simulink model "csdesigner_Preg_14v"  (R2014a)
settings: Solver=ode45  SolverMode=SingleTasking  StartTime=0.0  StopTime=10  RelTol=1e-3
values from neighbouring files (symbols this model uses):
  delay = 0.001    [init_regul.m]
  delta = 4e-6    (= 4e-06)    [main.m]
  Ecz = 0    [init_regul.m]
  F2 = a*mass*g/(a+b)    (= 15.4982642891)    [main.m]
  g = 9.81    [main.m]
  h0 = 75e-6    (= 7.5e-05)    [main.m]
  KAD = 0    [init_regul.m]
  Kpb = 5.5    [init_regul.m]
  Kps = (Vmax-Vmin)/(Hmax-Hmin)    (= 1666.66666667)    [main.m]
  Ksv = 30    [main.m]
  Kx = 1    [init_regul.m]
  Ky = 1    [init_regul.m]
  mm = F2/g    (= 1.57984345455)    [main.m]
  nu = 1/h0    (= 13333.3333333)    [main.m]
  omega = n_rpm*2*pi/60    (= 293.215314335)    [main.m]
  tau = 0.12    [main.m]
  Ts = 1/fs    (= 0.001)    [main.m]
  Ux0 = 3    [init_regul.m]
  Uy0 = 3    [init_regul.m]
  Wx = 5    [init_regul.m]
  Wy = 5    [init_regul.m]
  xeq = x(end,1)    [main.m]
  yeq = x(end,3)    [main.m]
undefined symbols (not defined in the file or in its folder): DiscIntNeverNeededParam
libraries: neural x162, dspmathops x4, simulink x3
(part 1 of 4)
settings Model: CovMetricSettings=dwe  CovHtmlReporting=off  covSaveCumulativeToWorkspaceVar=off  CovSaveSingleToWorkspaceVar=off  CovExternalEMLEnable=on  CovSFcnEnable=on  Creator=Alexander  LastModifiedBy=Юрий
settings DataIOCC: LimitDataPoints=off  SaveFormat=StructureWithTime  ReturnWorkspaceOutputs=on
settings DebuggingCC: MergeDetectMultiDrivingBlocksExec=error  SolverPrmCheckMsg=none  FrameProcessingCompatibilityMsg=error  SFUnexpectedBacktrackingDiag=error  SFNoUnconditionalDefaultTransitionDiag=error
settings HardwareCC: ProdBitPerPointer=64  ProdLargestAtomicFloat=Float  ProdIntDivRoundTo=Zero  ProdEndianess=LittleEndian  ProdHWDeviceType=Specified
settings ModelReferenceCC: PropagateSignalLabelsOutOfModel=on
settings SFSimCC: SimUseLocalCustomCode=on
settings RTWCC: RTWUseLocalCustomCode=on
settings GRTTargetCC: TargetLangStandard=C99 (ISO)

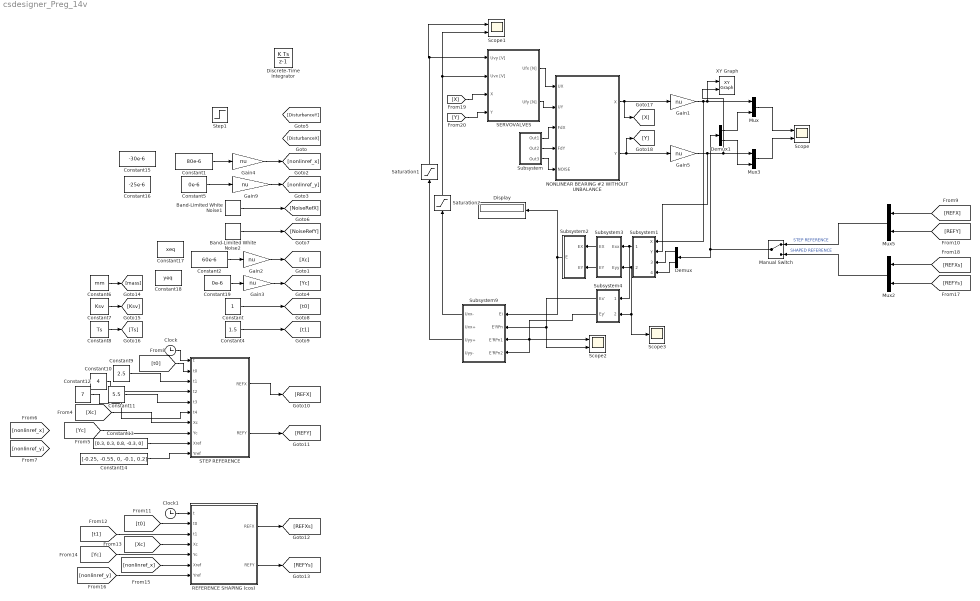
== system csdesigner_Preg_14v ==
  Band-Limited White Noise1 : simulink/Sources/Band-Limited White Noise  Cov=n_pow  Ts=Ts  seed=[23341]
  Band-Limited White Noise2 : simulink/Sources/Band-Limited White Noise  Cov=n_pow  Ts=1.1*Ts  seed=[23341]
  Clock : Clock
  Clock1 : Clock
  Constant : Constant
  Constant1 : Constant  Value=80e-6
  Constant10 : Constant  Value=4
  Constant11 : Constant  Value=5.5
  Constant12 : Constant  Value=7
  Constant13 : Constant  Value=[0.3, 0.3, 0.8, -0.3, 0]
  Constant14 : Constant  Value=[-0.25, -0.55, 0, -0.1, 0.2]
  Constant15 : Constant  Value=-30e-6
  Constant16 : Constant  Value=-25e-6
  Constant17 : Constant  Value=xeq
  Constant18 : Constant  Value=yeq
  Constant19 : Constant  Value=0e-6
  Constant2 : Constant  Value=60e-6
  Constant4 : Constant  Value=1.5
  Constant5 : Constant  Value=0e-6
  Constant6 : Constant  Value=mm
  Constant7 : Constant  Value=Ksv
  Constant8 : Constant  Value=Ts
  Constant9 : Constant  Value=2.5
  Demux : Demux  Outputs=2
  Demux1 : Demux  Outputs=2
  Discrete-Time Integrator : DiscreteIntegrator  InitialConditionSetting=State (most efficient)  SampleTime=-1  ICPrevOutput=DiscIntNeverNeededParam  ICPrevScaledInput=DiscIntNeverNeededParam
  Display : Display
  Gain{1..5,9} (6 alike) : Gain  Gain=nu
  Manual Switch : ManualSwitch
  Mux{,2..3,5} (4 alike) : Mux  Inputs=2
  NONLINEAR BEARING #2 WITHOUT UNBALANCE : Subsystem
  REFERENCE SHAPING (cos) : MATLAB Function  TreatAsAtomicUnit=on
      settings: PermitHierarchicalResolution=ParametersOnly
  SERVOVALVES : Subsystem
  STEP REFERENCE : MATLAB Function  TreatAsAtomicUnit=on
      settings: PermitHierarchicalResolution=ParametersOnly
  Saturation1 : Saturate  UpperLimit=10  LowerLimit=0
  Saturation2 : Saturate  UpperLimit=10  LowerLimit=0
  Scope : Scope  NumInputPorts=2
      settings: TimeRange=10  TickLabels=on  ShowLegends=on  MaxDataPoints=5000  SaveToWorkspace=off  SaveName=ScopeData  YMin=-0.50237~-0.65259  YMax=0.94471~0.29473  SampleTime=-1
  Scope1 : Scope  NumInputPorts=2
      settings: TimeRange=auto  MaxDataPoints=5000  SaveToWorkspace=off  YMin=-1.17846~-5  YMax=11.24205~5  SampleTime=-1
  Scope2 : Scope  NumInputPorts=2
      settings: TimeRange=auto  MaxDataPoints=5000  SaveToWorkspace=off  SaveName=ScopeData2  YMin=-1.34323~-5  YMax=0.95187~5  SampleTime=-1
  Scope3 : Scope
      settings: TimeRange=auto  MaxDataPoints=5000  SaveToWorkspace=off  SaveName=ScopeData2  YMin=-0.64553  YMax=0.24338  SampleTime=-1
  Step1 : Step  After=-10  SampleTime=0
  Subsystem : Subsystem
  Subsystem1 : Subsystem
  Subsystem2 : Subsystem
  Subsystem3 : Subsystem
  Subsystem4 : Subsystem
  Subsystem9 : Subsystem
  XY Graph : simulink/Sinks/XY Graph  xmin=-1  xmax=1  ymin=-1  ymax=1  st=-1
  wires:
  Constant7/1 -> [Ksv]
  [t0] -> STEP REFERENCE/2(t0)
  [nonlinref_y] -> REFERENCE SHAPING (cos)/7(Yref)
  [nonlinref_x] -> REFERENCE SHAPING (cos)/6(Xref)
  Constant8/1 -> [Ts]
  Constant6/1 -> [mass]
  Constant19/1 -> Gain3/1
  Mux5/1 -> Manual Switch/1  "STEP REFERENCE"
  [REFY] -> Mux5/2
  Clock1/1 -> REFERENCE SHAPING (cos)/1(t)
  Demux1/2 -> Mux3/2
  REFERENCE SHAPING (cos)/2(REFY) -> [REFYs]
  [REFX] -> Mux5/1
  Constant2/1 -> Gain2/1
  REFERENCE SHAPING (cos)/1(REFX) -> [REFXs]
  [Yc] -> REFERENCE SHAPING (cos)/5(Yc)
  Clock/1 -> STEP REFERENCE/1(t)
  [Xc] -> REFERENCE SHAPING (cos)/4(Xc)
  [t0] -> REFERENCE SHAPING (cos)/2(t0)
  Constant4/1 -> [t1]
  Gain3/1 -> [Yc]
  [REFXs] -> Mux2/1
  [t1] -> REFERENCE SHAPING (cos)/3(t1)
  [REFYs] -> Mux2/2
  [Xc] -> STEP REFERENCE/7(Xc)
  Mux2/1 -> Manual Switch/2  "SHAPED REFERENCE"
  Mux3/1 -> Scope/2
  Mux/1 -> Scope/1
  Manual Switch/1 -> Demux1/1, Demux/1
  STEP REFERENCE/2(REFY) -> [REFY]
  Gain4/1 -> [nonlinref_x]
  Gain2/1 -> [Xc]
  STEP REFERENCE/1(REFX) -> [REFX]
  Gain9/1 -> [nonlinref_y]
  [Yc] -> STEP REFERENCE/8(Yc)
  Constant5/1 -> Gain9/1
  Constant/1 -> [t0]
  NONLINEAR BEARING #2 WITHOUT UNBALANCE/1(X) -> [X], Gain1/1
  Band-Limited White Noise1/1 -> [NoiseRefX]
  Band-Limited White Noise2/1 -> [NoiseRefY]
  NONLINEAR BEARING #2 WITHOUT UNBALANCE/2(Y) -> [Y], Gain5/1
  Constant1/1 -> Gain4/1
  SERVOVALVES/1(Ufx [N]) -> NONLINEAR BEARING #2 WITHOUT UNBALANCE/1(UX)
  SERVOVALVES/2(Ufy [N]) -> NONLINEAR BEARING #2 WITHOUT UNBALANCE/2(UY)
  [X] -> SERVOVALVES/3(X)
  [Y] -> SERVOVALVES/4(Y)
  Gain1/1 -> Subsystem1/1(X), XY Graph/1, Mux/1
  Gain5/1 -> Subsystem1/2(Y), XY Graph/2, Mux3/1
  Subsystem/1(Out1) -> NONLINEAR BEARING #2 WITHOUT UNBALANCE/3(FdX)
  Subsystem/2(Out2) -> NONLINEAR BEARING #2 WITHOUT UNBALANCE/4(FdY)
  Subsystem/3(Out3) -> NONLINEAR BEARING #2 WITHOUT UNBALANCE/5(NOISE)
  Demux/1 -> Subsystem1/3(refX)
  Demux/2 -> Subsystem1/4(refY)
  Subsystem1/1(Exx) -> Subsystem4/1(Exx), Subsystem3/1(Exx)
  Subsystem3/1(EX) -> Subsystem2/1(EX)
  Subsystem1/2(Eyy) -> Scope3/1, Subsystem4/2(Eyy), Subsystem3/2(Eyy)
  Subsystem3/2(EY) -> Subsystem2/2(EY)
  Subsystem2/1(E) -> Subsystem9/1(Ei), Display/1
  Subsystem4/1(Ex') -> Subsystem9/2(E'RPn), Scope2/2
  Subsystem4/2(Ey') -> Subsystem9/4(E'RPn2), Scope2/1, Subsystem9/3(E'RPn1)
  Subsystem9/1(Uxx-) -> Saturation2/1
  Demux1/1 -> Mux/2
  Constant9/1 -> STEP REFERENCE/3(t1)
  Constant10/1 -> STEP REFERENCE/4(t2)
  Constant11/1 -> STEP REFERENCE/5(t3)
  Constant12/1 -> STEP REFERENCE/6(t4)
  Constant13/1 -> STEP REFERENCE/9(Xref)
  Constant14/1 -> STEP REFERENCE/10(Yref)
  Saturation1/1 -> Scope1/1, SERVOVALVES/1(Uvy [V])
  Saturation2/1 -> Scope1/2, SERVOVALVES/2(Uvx [V])
  Subsystem9/3(Uyy+) -> Saturation1/1

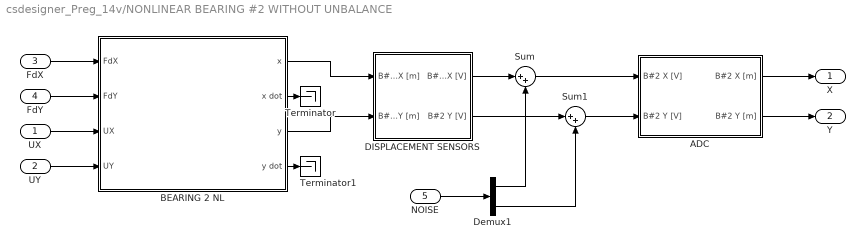
== system csdesigner_Preg_14v/NONLINEAR BEARING #2 WITHOUT UNBALANCE ==
  UX : Inport
  UY : Inport  Port=2
  FdX : Inport  Port=3
  FdY : Inport  Port=4
  NOISE : Inport  Port=5
  ADC : Subsystem
  BEARING 2 NL : Subsystem
  DISPLACEMENT SENSORS : Subsystem
  Demux1 : Demux  Outputs=2
  Sum : Sum  Inputs=|++
  Sum1 : Sum  Inputs=|++
  Terminator : Terminator
  Terminator1 : Terminator
  X : Outport
  Y : Outport  Port=2
  wires:
  BEARING 2 NL/3(y) -> DISPLACEMENT SENSORS/2(B#2 Y [m])
  BEARING 2 NL/1(x) -> DISPLACEMENT SENSORS/1(B#2 X [m])
  Demux1/2 -> Sum1/2
  NOISE/1 -> Demux1/1
  Demux1/1 -> Sum/2
  Sum1/1 -> ADC/2(B#2 Y [V])
  Sum/1 -> ADC/1(B#2 X [V])
  DISPLACEMENT SENSORS/1(B#2 X [V]) -> Sum/1
  DISPLACEMENT SENSORS/2(B#2 Y [V]) -> Sum1/1
  BEARING 2 NL/4(y dot) -> Terminator1/1
  BEARING 2 NL/2("x dot ") -> Terminator/1
  FdX/1 -> BEARING 2 NL/1(FdX)
  FdY/1 -> BEARING 2 NL/2(FdY)
  UY/1 -> BEARING 2 NL/4(UY)
  UX/1 -> BEARING 2 NL/3(UX)
  ADC/1(B#2 X [m]) -> X/1
  ADC/2(B#2 Y [m]) -> Y/1

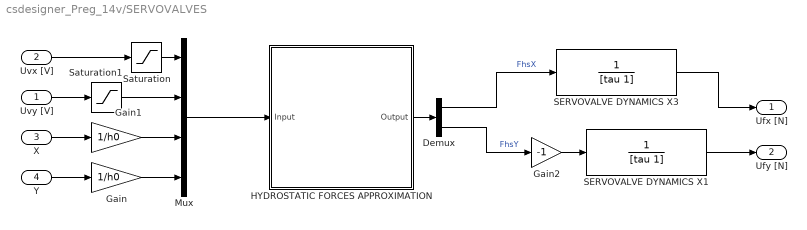
== system csdesigner_Preg_14v/SERVOVALVES ==
  Uvy [V] : Inport
  Uvx [V] : Inport  Port=2
  X : Inport  Port=3
  Y : Inport  Port=4
  Demux : Demux  Outputs=2
  Gain : Gain  Gain=1/h0
  Gain1 : Gain  Gain=1/h0
  Gain2 : Gain  Gain=-1
  HYDROSTATIC FORCES APPROXIMATION : Subsystem
      mask help: Function Fitting Neural Network
      mask Display: e = 0.06;c1 = [120 150 230]/255;c2 = ([120 150 230]+0)/383;c3 = ([120 150 230]+128)/383;patch([0 1 1 0],[0 0 1 1],c1);patch([0 1 1 1-e 1-e 0+e],[0 0 1 1-e 0+e 0+e],c2);patch([0 0 1 1-e 0+e 0+e],[0 1 1 1-e 1-e 0+e],c3);plot([0 1 1 0 0],[0 0 1 1 0]);fprintf('NNET');port_label('input',1,' Input');port_label('output',1,'Output ');
  Mux : Mux
  SERVOVALVE DYNAMICS X1 : TransferFcn  Numerator=1  Denominator=[tau 1]
  SERVOVALVE DYNAMICS X3 : TransferFcn  Numerator=1  Denominator=[tau 1]
  Saturation : Saturate  UpperLimit=10  LowerLimit=0
  Saturation1 : Saturate  UpperLimit=10  LowerLimit=0
  Ufx [N] : Outport
  Ufy [N] : Outport  Port=2
  wires:
  HYDROSTATIC FORCES APPROXIMATION/1(Output) -> Demux/1
  Demux/1 -> SERVOVALVE DYNAMICS X3/1  "FhsX"
  Demux/2 -> Gain2/1  "FhsY"
  Mux/1 -> HYDROSTATIC FORCES APPROXIMATION/1(Input)
  Y/1 -> Gain/1
  X/1 -> Gain1/1
  Uvy [V]/1 -> Saturation1/1
  Uvx [V]/1 -> Saturation/1
  Gain/1 -> Mux/4
  Gain1/1 -> Mux/3
  Saturation/1 -> Mux/1
  Saturation1/1 -> Mux/2
  Gain2/1 -> SERVOVALVE DYNAMICS X1/1
  SERVOVALVE DYNAMICS X3/1 -> Ufx [N]/1
  SERVOVALVE DYNAMICS X1/1 -> Ufy [N]/1

== system csdesigner_Preg_14v/Subsystem ==
  Mux1 : Mux  Inputs=2
  Out1 : Outport
  Out2 : Outport  Port=2
  Out3 : Outport  Port=3
  wires:
  [NoiseRefY] -> Mux1/2
  [NoiseRefX] -> Mux1/1
  [DisturbanceX] -> Out1/1
  [DisturbanceY] -> Out2/1
  Mux1/1 -> Out3/1

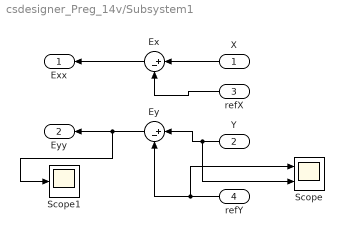
== system csdesigner_Preg_14v/Subsystem1 ==
  X : Inport
  Y : Inport  Port=2
  refX : Inport  Port=3
  refY : Inport  Port=4
  Ex : Sum  Inputs=|+-
  Ey : Sum  Inputs=|+-
  Scope : Scope  NumInputPorts=2
      settings: TimeRange=auto  MaxDataPoints=5000  SaveToWorkspace=off  SaveName=ScopeData3  YMin=-0.65259~-5  YMax=0.29473~5  SampleTime=-1
  Scope1 : Scope
      settings: TimeRange=auto  MaxDataPoints=5000  SaveToWorkspace=off  SaveName=ScopeData4  YMin=-0.64553  YMax=0.24338  SampleTime=-1
  Exx : Outport
  Eyy : Outport  Port=2
  wires:
  Ex/1 -> Exx/1
  Ey/1 -> Scope1/1, Eyy/1
  refX/1 -> Ex/2
  X/1 -> Ex/1
  Y/1 -> Scope/2, Ey/1
  refY/1 -> Scope/1, Ey/2

== system csdesigner_Preg_14v/Subsystem2 ==
  EX : Inport
  EY : Inport  Port=2
  Math Function : Math  Operator=square  SaturateOnIntegerOverflow=on
  Math Function1 : Math  Operator=square  SaturateOnIntegerOverflow=on
  Sqrt : Sqrt  SaturateOnIntegerOverflow=on
  Sum : Sum  Inputs=|++
  E : Outport
  wires:
  Sum/1 -> Sqrt/1
  Math Function1/1 -> Sum/2
  Math Function/1 -> Sum/1
  EY/1 -> Math Function1/1
  EX/1 -> Math Function/1
  Sqrt/1 -> E/1

== system csdesigner_Preg_14v/Subsystem3 ==
  Exx : Inport
  Eyy : Inport  Port=2
  Constant9 : Constant  Value=Ecz
  Sum : Sum  Inputs=|++
  Sum1 : Sum  Inputs=|++
  EX : Outport
  EY : Outport  Port=2
  wires:
  Constant9/1 -> Sum/2, Sum1/2
  Sum/1 -> EX/1
  Eyy/1 -> Sum1/1
  Sum1/1 -> EY/1
  Exx/1 -> Sum/1

== system csdesigner_Preg_14v/Subsystem4 ==
  Exx : Inport
  Eyy : Inport  Port=2
  Constant9 : Constant  Value=Ecz
  Sum : Sum  Inputs=|+-
  Sum1 : Sum  Inputs=|+-
  Ex' : Outport
  Ey' : Outport  Port=2
  wires:
  Constant9/1 -> Sum/2, Sum1/2
  Exx/1 -> Sum/1
  Eyy/1 -> Sum1/1
  Sum1/1 -> Ey'/1
  Sum/1 -> Ex'/1

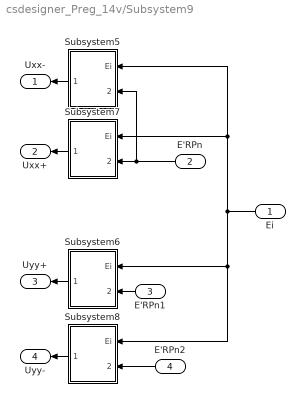
== system csdesigner_Preg_14v/Subsystem9 ==
  Ei : Inport
  E'RPn : Inport  Port=2
  E'RPn1 : Inport  Port=3
  E'RPn2 : Inport  Port=4
  Subsystem5 : Subsystem
  Subsystem6 : Subsystem
  Subsystem7 : Subsystem
  Subsystem8 : Subsystem
  Uxx- : Outport
  Uxx+ : Outport  Port=2
  Uyy+ : Outport  Port=3
  Uyy- : Outport  Port=4
  wires:
  Ei/1 -> Subsystem7/1(Ei), Subsystem5/1(Ei), Subsystem6/1(Ei), Subsystem8/1(Ei)
  E'RPn/1 -> Subsystem7/2(E'RPn), Subsystem5/2(E'RPn)
  E'RPn2/1 -> Subsystem8/2(E'RPn)
  Subsystem6/1(Uyy+) -> Uyy+/1
  Subsystem5/1(Uxx-) -> Uxx-/1
  Subsystem7/1(Uxx+) -> Uxx+/1
  E'RPn1/1 -> Subsystem6/2(E'RPn)
  Subsystem8/1(Uyy-) -> Uyy-/1

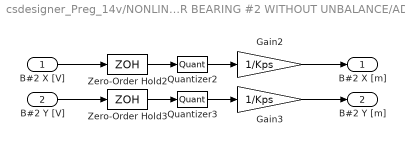
== system csdesigner_Preg_14v/NONLINEAR BEARING #2 WITHOUT UNBALANCE/ADC ==
  B#2 X [V] : Inport
  B#2 Y [V] : Inport  Port=2
  Gain2 : Gain  Gain=1/Kps
  Gain3 : Gain  Gain=1/Kps
  Quantizer2 : Quantizer  QuantizationInterval=0.000152587890625
  Quantizer3 : Quantizer  QuantizationInterval=0.000152587890625
  Zero-Order Hold2 : ZeroOrderHold  SampleTime=Ts
  Zero-Order Hold3 : ZeroOrderHold  SampleTime=Ts
  B#2 X [m] : Outport
  B#2 Y [m] : Outport  Port=2
  wires:
  B#2 Y [V]/1 -> Zero-Order Hold3/1
  Zero-Order Hold3/1 -> Quantizer3/1
  Gain3/1 -> B#2 Y [m]/1
  Zero-Order Hold2/1 -> Quantizer2/1
  Gain2/1 -> B#2 X [m]/1
  B#2 X [V]/1 -> Zero-Order Hold2/1
  Quantizer3/1 -> Gain3/1
  Quantizer2/1 -> Gain2/1

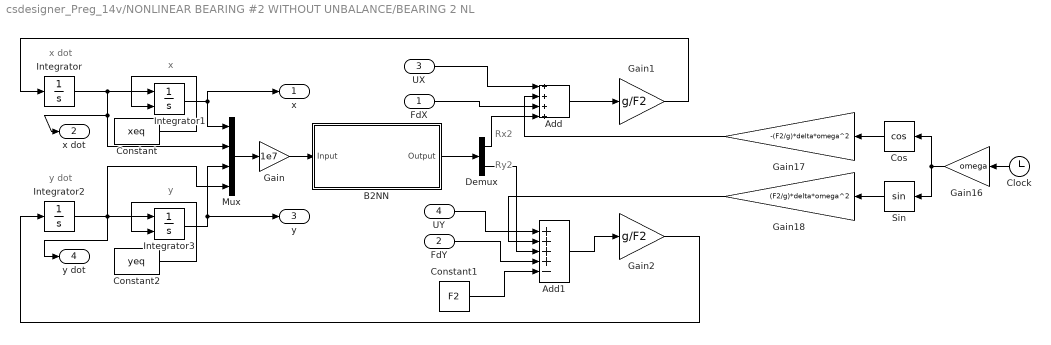
== system csdesigner_Preg_14v/NONLINEAR BEARING #2 WITHOUT UNBALANCE/BEARING 2 NL ==
  note: x
  note: x dot
  note: y
  note: y dot
  note: Ry2
  note: Rx2
  FdX : Inport
  FdY : Inport  Port=2
  UX : Inport  Port=3
  UY : Inport  Port=4
  Add : Sum  Inputs=++++
  Add1 : Sum  Inputs=++++-
  "B2NN " : Subsystem
      mask help: Feed-Forward Neural Network
      mask Display: e = 0.06;c1 = [120 150 230]/255;c2 = ([120 150 230]+0)/383;c3 = ([120 150 230]+128)/383;patch([0 1 1 0],[0 0 1 1],c1);patch([0 1 1 1-e 1-e 0+e],[0 0 1 1-e 0+e 0+e],c2);patch([0 0 1 1-e 0+e 0+e],[0 1 1 1-e 1-e 0+e],c3);plot([0 1 1 0 0],[0 0 1 1 0]);fprintf('B2 NNET');port_label('input',1,' X');port_label('output',1,'F ');
  Clock : Clock
  Constant : Constant  Value=xeq
  Constant1 : Constant  Value=F2
  Constant2 : Constant  Value=yeq
  Cos : Trigonometry  Operator=cos
  Demux : Demux  Outputs=2
  Gain : Gain  Gain=1e7
  Gain1 : Gain  Gain=g/F2
  Gain16 : Gain  Gain=omega
  Gain17 : Gain  Gain=-(F2/g)*delta*omega^2
  Gain18 : Gain  Gain=(F2/g)*delta*omega^2
  Gain2 : Gain  Gain=g/F2
  Integrator : Integrator
  Integrator1 : Integrator  InitialConditionSource=external  InitialCondition=-14.8e-6
  Integrator2 : Integrator
  Integrator3 : Integrator  InitialConditionSource=external  InitialCondition=-4.41e-6
  Mux : Mux
  Sin : Trigonometry
  x : Outport
  "x dot " : Outport  Port=2
  y : Outport  Port=3
  y dot : Outport  Port=4
  wires:
  Add1/1 -> Gain2/1
  Gain1/1 -> Integrator/1
  FdY/1 -> Add1/4
  Integrator/1 -> Mux/2, "x dot "/1, Integrator1/1
  Integrator1/1 -> x/1, Mux/1
  Integrator2/1 -> y dot/1, Mux/4, Integrator3/1
  Add/1 -> Gain1/1
  Integrator3/1 -> y/1, Mux/3
  FdX/1 -> Add/3
  Mux/1 -> Gain/1
  Demux/2 -> Add1/3
  Gain/1 -> "B2NN "/1(Input)
  Demux/1 -> Add/4
  Gain2/1 -> Integrator2/1
  Constant1/1 -> Add1/5
  "B2NN "/1(Output) -> Demux/1
  UX/1 -> Add/1
  UY/1 -> Add1/1
  Constant/1 -> Integrator1/2
  Constant2/1 -> Integrator3/2
  Clock/1 -> Gain16/1
  Cos/1 -> Gain17/1
  Sin/1 -> Gain18/1
  Gain16/1 -> Sin/1, Cos/1
  Gain18/1 -> Add1/2
  Gain17/1 -> Add/2

== system csdesigner_Preg_14v/NONLINEAR BEARING #2 WITHOUT UNBALANCE/DISPLACEMENT SENSORS ==
  B#2 X [m] : Inport
  B#2 Y [m] : Inport  Port=2
  Gain : Gain  Gain=Kps
  Gain1 : Gain  Gain=Kps
  B#2 X [V] : Outport
  B#2 Y [V] : Outport  Port=2
  wires:
  Gain1/1 -> B#2 Y [V]/1
  Gain/1 -> B#2 X [V]/1
  B#2 X [m]/1 -> Gain/1
  B#2 Y [m]/1 -> Gain1/1

== system csdesigner_Preg_14v/SERVOVALVES/HYDROSTATIC FORCES APPROXIMATION ==
  Input : Inport  PortDimensions=4
      mask Display: e = 0.06;c1 = [120 230 180]/255;c2 = ([120 230 180]+0)/(256+128);c3 = ([120 230 180]+128)/(256+128);patch([0 1 1 0],[0 0 1 1],c1);patch([0 1 1 1-e 1-e 0+e],[0 0 1 1-e 0+e 0+e],c2);patch([0 0 1 1-e 0+e 0+e],[0 1 1 1-e 1-e 0+e],c3);plot([0 1 1 0 0],[0 0 1 1 0]);
  Layer 1 : Subsystem
      mask Display: e = 0.06;c1 = [120 150 230]/255;c2 = ([120 150 230]+0)/383;c3 = ([120 150 230]+128)/383;patch([0 1 1 0],[0 0 1 1],c1);patch([0 1 1 1-e 1-e 0+e],[0 0 1 1-e 0+e 0+e],c2);patch([0 0 1 1-e 0+e 0+e],[0 1 1 1-e 1-e 0+e],c3);plot([0 1 1 0 0],[0 0 1 1 0]);
  Layer 2 : Subsystem
      mask Display: e = 0.06;c1 = [120 150 230]/255;c2 = ([120 150 230]+0)/383;c3 = ([120 150 230]+128)/383;patch([0 1 1 0],[0 0 1 1],c1);patch([0 1 1 1-e 1-e 0+e],[0 0 1 1-e 0+e 0+e],c2);patch([0 0 1 1-e 0+e 0+e],[0 1 1 1-e 1-e 0+e],c3);plot([0 1 1 0 0],[0 0 1 1 0]);
  Process Input 1 : Subsystem
      mask Display: e = 0.06;c1 = [120 150 230]/255;c2 = ([120 150 230]+0)/383;c3 = ([120 150 230]+128)/383;patch([0 1 1 0],[0 0 1 1],c1);patch([0 1 1 1-e 1-e 0+e],[0 0 1 1-e 0+e 0+e],c2);patch([0 0 1 1-e 0+e 0+e],[0 1 1 1-e 1-e 0+e],c3);plot([0 1 1 0 0],[0 0 1 1 0]);
  Process Output 1 : Subsystem
      mask Display: e = 0.06;c1 = [120 150 230]/255;c2 = ([120 150 230]+0)/383;c3 = ([120 150 230]+128)/383;patch([0 1 1 0],[0 0 1 1],c1);patch([0 1 1 1-e 1-e 0+e],[0 0 1 1-e 0+e 0+e],c2);patch([0 0 1 1-e 0+e 0+e],[0 1 1 1-e 1-e 0+e],c3);plot([0 1 1 0 0],[0 0 1 1 0]);
  Output : Outport  InitialOutput=[0;0]
      mask Display: e = 0.06;c1 = [120 230 180]/255;c2 = ([120 230 180]+0)/(256+128);c3 = ([120 230 180]+128)/(256+128);patch([0 1 1 0],[0 0 1 1],c1);patch([0 1 1 1-e 1-e 0+e],[0 0 1 1-e 0+e 0+e],c2);patch([0 0 1 1-e 0+e 0+e],[0 1 1 1-e 1-e 0+e],c3);plot([0 1 1 0 0],[0 0 1 1 0]);
  wires:
  Input/1 -> Process Input 1/1(x)
  Process Output 1/1(y) -> Output/1
  Process Input 1/1(p) -> Layer 1/1("p{1}")
  Layer 1/1("a{1}") -> [feedback1]
  [feedback1] -> Layer 2/1("a{1} ")
  Layer 2/1("a{2}") -> Process Output 1/1(a)

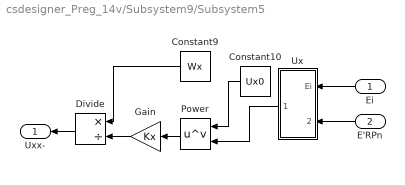
== system csdesigner_Preg_14v/Subsystem9/Subsystem5 ==
  Ei : Inport
  E'RPn : Inport  Port=2
  Constant10 : Constant  Value=Ux0
  Constant9 : Constant  Value=Wx
  Divide : Product  Inputs=*/
  Gain : Gain  Gain=Kx
  Power : Math  Operator=pow  SaturateOnIntegerOverflow=on
  Ux : Subsystem
  Uxx- : Outport
  wires:
  Divide/1 -> Uxx-/1
  Constant9/1 -> Divide/1
  Power/1 -> Gain/1
  Constant10/1 -> Power/1
  Ei/1 -> Ux/1(Ei)
  E'RPn/1 -> Ux/2(E'RPn)
  Ux/1(Ux) -> Power/2
  Gain/1 -> Divide/2

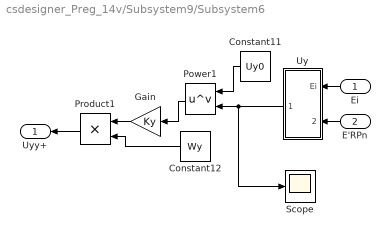
== system csdesigner_Preg_14v/Subsystem9/Subsystem6 ==
  Ei : Inport
  E'RPn : Inport  Port=2
  Constant11 : Constant  Value=Uy0
  Constant12 : Constant  Value=Wy
  Gain : Gain  Gain=Ky
  Power1 : Math  Operator=pow  SaturateOnIntegerOverflow=on
  Product1 : Product
  Scope : Scope
      settings: TimeRange=auto  MaxDataPoints=5000  SaveToWorkspace=off  YMin=-3.55043  YMax=1.33861  SampleTime=-1
  Uy : Subsystem
  Uyy+ : Outport
  wires:
  Constant11/1 -> Power1/1
  Power1/1 -> Gain/1
  Ei/1 -> Uy/1(Ei)
  Product1/1 -> Uyy+/1
  Constant12/1 -> Product1/2
  E'RPn/1 -> Uy/2(E'RPn)
  Uy/1(Uy) -> Scope/1, Power1/2
  Gain/1 -> Product1/1

== system csdesigner_Preg_14v/Subsystem9/Subsystem7 ==
  Ei : Inport
  E'RPn : Inport  Port=2
  Constant10 : Constant  Value=Ux0
  Constant9 : Constant  Value=Wx
  Gain : Gain  Gain=Kx
  Power : Math  Operator=pow  SaturateOnIntegerOverflow=on
  Product : Product
  Ux : Subsystem
  Uxx+ : Outport
  wires:
  Product/1 -> Uxx+/1
  Constant9/1 -> Product/1
  Power/1 -> Gain/1
  Constant10/1 -> Power/1
  Ei/1 -> Ux/1(Ei)
  E'RPn/1 -> Ux/2(E'RPn)
  Ux/1(Ux) -> Power/2
  Gain/1 -> Product/2

== system csdesigner_Preg_14v/Subsystem9/Subsystem8 ==
  Ei : Inport
  E'RPn : Inport  Port=2
  Constant11 : Constant  Value=Uy0
  Constant12 : Constant  Value=Wy
  Divide : Product  Inputs=*/
  Gain : Gain  Gain=Ky
  Power1 : Math  Operator=pow  SaturateOnIntegerOverflow=on
  Uy : Subsystem
  Uyy- : Outport
  wires:
  Constant11/1 -> Power1/1
  Power1/1 -> Gain/1
  Ei/1 -> Uy/1(Ei)
  Divide/1 -> Uyy-/1
  Constant12/1 -> Divide/1
  E'RPn/1 -> Uy/2(E'RPn)
  Uy/1(Uy) -> Power1/2
  Gain/1 -> Divide/2

== system csdesigner_Preg_14v/NONLINEAR BEARING #2 WITHOUT UNBALANCE/BEARING 2 NL/B2NN  ==
  Input : Inport  PortDimensions=4
      mask Display: e = 0.06;c1 = [120 230 180]/255;c2 = ([120 230 180]+0)/(256+128);c3 = ([120 230 180]+128)/(256+128);patch([0 1 1 0],[0 0 1 1],c1);patch([0 1 1 1-e 1-e 0+e],[0 0 1 1-e 0+e 0+e],c2);patch([0 0 1 1-e 0+e 0+e],[0 1 1 1-e 1-e 0+e],c3);plot([0 1 1 0 0],[0 0 1 1 0]);
  Layer 1 : Subsystem
      mask Display: e = 0.06;c1 = [120 150 230]/255;c2 = ([120 150 230]+0)/383;c3 = ([120 150 230]+128)/383;patch([0 1 1 0],[0 0 1 1],c1);patch([0 1 1 1-e 1-e 0+e],[0 0 1 1-e 0+e 0+e],c2);patch([0 0 1 1-e 0+e 0+e],[0 1 1 1-e 1-e 0+e],c3);plot([0 1 1 0 0],[0 0 1 1 0]);
  Layer 2 : Subsystem
      mask Display: e = 0.06;c1 = [120 150 230]/255;c2 = ([120 150 230]+0)/383;c3 = ([120 150 230]+128)/383;patch([0 1 1 0],[0 0 1 1],c1);patch([0 1 1 1-e 1-e 0+e],[0 0 1 1-e 0+e 0+e],c2);patch([0 0 1 1-e 0+e 0+e],[0 1 1 1-e 1-e 0+e],c3);plot([0 1 1 0 0],[0 0 1 1 0]);
  Process Input 1 : Subsystem
      mask Display: e = 0.06;c1 = [120 150 230]/255;c2 = ([120 150 230]+0)/383;c3 = ([120 150 230]+128)/383;patch([0 1 1 0],[0 0 1 1],c1);patch([0 1 1 1-e 1-e 0+e],[0 0 1 1-e 0+e 0+e],c2);patch([0 0 1 1-e 0+e 0+e],[0 1 1 1-e 1-e 0+e],c3);plot([0 1 1 0 0],[0 0 1 1 0]);
  Process Output 1 : Subsystem
      mask Display: e = 0.06;c1 = [120 150 230]/255;c2 = ([120 150 230]+0)/383;c3 = ([120 150 230]+128)/383;patch([0 1 1 0],[0 0 1 1],c1);patch([0 1 1 1-e 1-e 0+e],[0 0 1 1-e 0+e 0+e],c2);patch([0 0 1 1-e 0+e 0+e],[0 1 1 1-e 1-e 0+e],c3);plot([0 1 1 0 0],[0 0 1 1 0]);
  Output : Outport  InitialOutput=[0;0]
      mask Display: e = 0.06;c1 = [120 230 180]/255;c2 = ([120 230 180]+0)/(256+128);c3 = ([120 230 180]+128)/(256+128);patch([0 1 1 0],[0 0 1 1],c1);patch([0 1 1 1-e 1-e 0+e],[0 0 1 1-e 0+e 0+e],c2);patch([0 0 1 1-e 0+e 0+e],[0 1 1 1-e 1-e 0+e],c3);plot([0 1 1 0 0],[0 0 1 1 0]);
  wires:
  Input/1 -> Process Input 1/1(x)
  Process Output 1/1(y) -> Output/1
  Process Input 1/1(p) -> Layer 1/1("p{1}")
  Layer 1/1("a{1}") -> [feedback1]
  [feedback1] -> Layer 2/1("a{1} ")
  Layer 2/1("a{2}") -> Process Output 1/1(a)

== system csdesigner_Preg_14v/SERVOVALVES/HYDROSTATIC FORCES APPROXIMATION/Layer 1 ==
  "p{1}" : Inport  PortDimensions=4
      mask Display: e = 0.06;c1 = [120 230 180]/255;c2 = ([120 230 180]+0)/(256+128);c3 = ([120 230 180]+128)/(256+128);patch([0 1 1 0],[0 0 1 1],c1);patch([0 1 1 1-e 1-e 0+e],[0 0 1 1-e 0+e 0+e],c2);patch([0 0 1 1-e 0+e 0+e],[0 1 1 1-e 1-e 0+e],c3);plot([0 1 1 0 0],[0 0 1 1 0]);
  Delays 1 : Subsystem
      mask Display: e = 0.06;c1 = [120 150 230]/255;c2 = ([120 150 230]+0)/383;c3 = ([120 150 230]+128)/383;patch([0 1 1 0],[0 0 1 1],c1);patch([0 1 1 1-e 1-e 0+e],[0 0 1 1-e 0+e 0+e],c2);patch([0 0 1 1-e 0+e 0+e],[0 1 1 1-e 1-e 0+e],c3);plot([0 1 1 0 0],[0 0 1 1 0]);disp('0');
  "IW{1,1}" : Subsystem
      mask Display: e = 0.06;c1 = [120 150 230]/255;c2 = ([120 150 230]+0)/383;c3 = ([120 150 230]+128)/383;patch([0 1 1 0],[0 0 1 1],c1);patch([0 1 1 1-e 1-e 0+e],[0 0 1 1-e 0+e 0+e],c2);patch([0 0 1 1-e 0+e 0+e],[0 1 1 1-e 1-e 0+e],c3);plot([0 1 1 0 0],[0 0 1 1 0]);disp('W');
  "b{1}" : Constant  Value=[-0.23296643016029394690491471919813193380832672119140625;0.326049712013471271188080891079152934253215789794921875;0.7635980530113568587324834879836998879909515380859375;0.0371341804022077559555015113801346160471439361572265625;1.48461274019036881810507111367769539356231689453125;-0.77588780174378013665403841514489613473415374755859375;0.1053125860621959841711969829702866263687610626220703125;1.0298649297191155849162669255747459828853607177734375;-1.3892844353472038054775339332991279661655426025390625;0.2077419320335334995686338288578554056584835052490234375;2.455823784380505525604121430660597980022430419921875;-1.042792187924732605353028702666051685810089111328125;-0.83741911975379312860212621671962551772594451904296875;-0.63813908685641773654850794628146104514598846435546875;1.3804994976031419451345527704688720405101776123046875;1.6260889286423421129512689731200225651264190673828125;-0.037184626673177741118525574393061106093227863311767578125;-0.06924958740920213184910636528002214618027210235595703125;0.3874880326547402997761082588112913072109222412109375;-0.319507389127828000940922947847866453230381011962890625;-0.10898018603528909775679522908831131644546985626220703125;1.9920530318482303488991647100192494690418243408203125;-0.87367561016282480057526527161826379597187042236328125;-0.0160003355843557799886855974591526319272816181182861328125;-0.365573385995172583928791709695360623300075531005859375;-0.441160874329397600934754564150352962315082550048828125;-0.292666719397117469636526720933034084737300872802734375;0.1229263675405330713541474096928141079843044281005859375;0.04745390456252561450778415519380359910428524017333984375;-0.035143918645035417125388477188607794232666492462158203125;0.388770231468412885700303149860701523721218109130859375;0.23016135712277996372421284831943921744823455810546875;0.2215605353991782766609475174846011213958263397216796875;0.7662017223235941809633686716551892459392547607421875;0.90362072723460451495469669680460356175899505615234375;0.8761600354448766392323477703030221164226531982421875;-0.6860324553056178498167128054774366319179534912109375;-0.435376129942828260510623294976539909839630126953125;-0.3066151492141153678261389359249733388423919677734375;0.5722836445991574816360980548779480159282684326171875;0.1905023414738137577106869002818712033331394195556640625;-0.1122246052501608415408185237538418732583522796630859375;1.7151489516827316261782243600464425981044769287109375;-0.26475416583770339240544444692204706370830535888671875;-0.988047096077767417199311239528469741344451904296875;-2.6764998664684060969420897890813648700714111328125;4.7795834629228775014553320943377912044525146484375;1.7458993710812944488708353674155659973621368408203125;1.1453040148301003586794877264765091240406036376953125;0.82241561116589856350600484802271239459514617919921875]
      mask Display: e = 0.06;c1 = [120 150 230]/255;c2 = ([120 150 230]+0)/383;c3 = ([120 150 230]+128)/383;patch([0 1 1 0],[0 0 1 1],c1);patch([0 1 1 1-e 1-e 0+e],[0 0 1 1-e 0+e 0+e],c2);patch([0 0 1 1-e 0+e 0+e],[0 1 1 1-e 1-e 0+e],c3);plot([0 1 1 0 0],[0 0 1 1 0]);disp('b');
  netsum : Sum  Inputs=2  InputSameDT=on  SaturateOnIntegerOverflow=on  OutDataTypeStr=Inherit: Same as first input
      mask Display: e = 0.06;c1 = [120 150 230]/255;c2 = ([120 150 230]+0)/383;c3 = ([120 150 230]+128)/383;patch([0 1 1 0],[0 0 1 1],c1);patch([0 1 1 1-e 1-e 0+e],[0 0 1 1-e 0+e 0+e],c2);patch([0 0 1 1-e 0+e 0+e],[0 1 1 1-e 1-e 0+e],c3);plot([0 1 1 0 0],[0 0 1 1 0]);disp('+');
  tansig : neural/Transfer Functions/tansig
  "a{1}" : Outport  InitialOutput=[0;0;0;0;0;0;0;0;0;0;0;0;0;0;0;0;0;0;0;0;0;0;0;0;0;0;0;0;0;0;0;0;0;0;0;0;0;0;0;0;0;0;0;0;0;0;0;0;0;0]
      mask Display: e = 0.06;c1 = [120 230 180]/255;c2 = ([120 230 180]+0)/(256+128);c3 = ([120 230 180]+128)/(256+128);patch([0 1 1 0],[0 0 1 1],c1);patch([0 1 1 1-e 1-e 0+e],[0 0 1 1-e 0+e 0+e],c2);patch([0 0 1 1-e 0+e 0+e],[0 1 1 1-e 1-e 0+e],c3);plot([0 1 1 0 0],[0 0 1 1 0]);
  wires:
  "p{1}"/1 -> Delays 1/1("p{1}")
  Delays 1/1("pd{1,1}") -> "IW{1,1}"/1("pd{1,1}")
  "IW{1,1}"/1("iz{1,1}") -> netsum/1
  "b{1}"/1 -> netsum/2
  netsum/1 -> tansig/1
  tansig/1 -> "a{1}"/1

== system csdesigner_Preg_14v/SERVOVALVES/HYDROSTATIC FORCES APPROXIMATION/Layer 2 ==
  "a{1} " : Inport  PortDimensions=50
      mask Display: e = 0.06;c1 = [120 230 180]/255;c2 = ([120 230 180]+0)/(256+128);c3 = ([120 230 180]+128)/(256+128);patch([0 1 1 0],[0 0 1 1],c1);patch([0 1 1 1-e 1-e 0+e],[0 0 1 1-e 0+e 0+e],c2);patch([0 0 1 1-e 0+e 0+e],[0 1 1 1-e 1-e 0+e],c3);plot([0 1 1 0 0],[0 0 1 1 0]);
  Delays 1 : Subsystem
      mask Display: e = 0.06;c1 = [120 150 230]/255;c2 = ([120 150 230]+0)/383;c3 = ([120 150 230]+128)/383;patch([0 1 1 0],[0 0 1 1],c1);patch([0 1 1 1-e 1-e 0+e],[0 0 1 1-e 0+e 0+e],c2);patch([0 0 1 1-e 0+e 0+e],[0 1 1 1-e 1-e 0+e],c3);plot([0 1 1 0 0],[0 0 1 1 0]);disp('0');
  "LW{2,1}" : Subsystem
      mask Display: e = 0.06;c1 = [120 150 230]/255;c2 = ([120 150 230]+0)/383;c3 = ([120 150 230]+128)/383;patch([0 1 1 0],[0 0 1 1],c1);patch([0 1 1 1-e 1-e 0+e],[0 0 1 1-e 0+e 0+e],c2);patch([0 0 1 1-e 0+e 0+e],[0 1 1 1-e 1-e 0+e],c3);plot([0 1 1 0 0],[0 0 1 1 0]);disp('W');
  "b{2}" : Constant  Value=[-0.9133793217564865063451406967942602932453155517578125;0.5937312331962754097247625395539216697216033935546875]
      mask Display: e = 0.06;c1 = [120 150 230]/255;c2 = ([120 150 230]+0)/383;c3 = ([120 150 230]+128)/383;patch([0 1 1 0],[0 0 1 1],c1);patch([0 1 1 1-e 1-e 0+e],[0 0 1 1-e 0+e 0+e],c2);patch([0 0 1 1-e 0+e 0+e],[0 1 1 1-e 1-e 0+e],c3);plot([0 1 1 0 0],[0 0 1 1 0]);disp('b');
  netsum : Sum  Inputs=2  InputSameDT=on  SaturateOnIntegerOverflow=on  OutDataTypeStr=Inherit: Same as first input
      mask Display: e = 0.06;c1 = [120 150 230]/255;c2 = ([120 150 230]+0)/383;c3 = ([120 150 230]+128)/383;patch([0 1 1 0],[0 0 1 1],c1);patch([0 1 1 1-e 1-e 0+e],[0 0 1 1-e 0+e 0+e],c2);patch([0 0 1 1-e 0+e 0+e],[0 1 1 1-e 1-e 0+e],c3);plot([0 1 1 0 0],[0 0 1 1 0]);disp('+');
  purelin : neural/Transfer Functions/purelin
  "a{2}" : Outport  InitialOutput=[0;0]
      mask Display: e = 0.06;c1 = [120 230 180]/255;c2 = ([120 230 180]+0)/(256+128);c3 = ([120 230 180]+128)/(256+128);patch([0 1 1 0],[0 0 1 1],c1);patch([0 1 1 1-e 1-e 0+e],[0 0 1 1-e 0+e 0+e],c2);patch([0 0 1 1-e 0+e 0+e],[0 1 1 1-e 1-e 0+e],c3);plot([0 1 1 0 0],[0 0 1 1 0]);
  wires:
  "a{1} "/1 -> Delays 1/1("p{2}")
  Delays 1/1("pd{2,1}") -> "LW{2,1}"/1("ad{2,1}")
  "LW{2,1}"/1("lz{2,1}") -> netsum/1
  "b{2}"/1 -> netsum/2
  netsum/1 -> purelin/1
  purelin/1 -> "a{2}"/1

== system csdesigner_Preg_14v/SERVOVALVES/HYDROSTATIC FORCES APPROXIMATION/Process Input 1 ==
  x : Inport  PortDimensions=4
      mask Display: e = 0.06;c1 = [120 230 180]/255;c2 = ([120 230 180]+0)/(256+128);c3 = ([120 230 180]+128)/(256+128);patch([0 1 1 0],[0 0 1 1],c1);patch([0 1 1 1-e 1-e 0+e],[0 0 1 1-e 0+e 0+e],c2);patch([0 0 1 1-e 0+e 0+e],[0 1 1 1-e 1-e 0+e],c3);plot([0 1 1 0 0],[0 0 1 1 0]);
  mapminmax : neural/Processing Functions/mapminmax  xmin=[0;0;-0.900000000000000022204460492503;-0.900000000000000022204460492503]  xmax=[10;10;0.900000000000000022204460492503;0.900000000000000022204460492503]  ymin=-1  ymax=1
  p : Outport  PortDimensions=4
      mask Display: e = 0.06;c1 = [120 230 180]/255;c2 = ([120 230 180]+0)/(256+128);c3 = ([120 230 180]+128)/(256+128);patch([0 1 1 0],[0 0 1 1],c1);patch([0 1 1 1-e 1-e 0+e],[0 0 1 1-e 0+e 0+e],c2);patch([0 0 1 1-e 0+e 0+e],[0 1 1 1-e 1-e 0+e],c3);plot([0 1 1 0 0],[0 0 1 1 0]);
  wires:
  x/1 -> mapminmax/1
  mapminmax/1 -> p/1

== system csdesigner_Preg_14v/SERVOVALVES/HYDROSTATIC FORCES APPROXIMATION/Process Output 1 ==
  a : Inport  PortDimensions=2
      mask Display: e = 0.06;c1 = [120 230 180]/255;c2 = ([120 230 180]+0)/(256+128);c3 = ([120 230 180]+128)/(256+128);patch([0 1 1 0],[0 0 1 1],c1);patch([0 1 1 1-e 1-e 0+e],[0 0 1 1-e 0+e 0+e],c2);patch([0 0 1 1-e 0+e 0+e],[0 1 1 1-e 1-e 0+e],c3);plot([0 1 1 0 0],[0 0 1 1 0]);
  mapminmax_reverse : neural/Processing Functions/mapminmax_reverse  xmin=[-39.2059127735752639409838593565;-44.6541129541421923931920900941]  xmax=[54.8807190337208083974473993294;75.0887247836675868484235252254]  ymin=-1  ymax=1
  y : Outport  PortDimensions=2
      mask Display: e = 0.06;c1 = [120 230 180]/255;c2 = ([120 230 180]+0)/(256+128);c3 = ([120 230 180]+128)/(256+128);patch([0 1 1 0],[0 0 1 1],c1);patch([0 1 1 1-e 1-e 0+e],[0 0 1 1-e 0+e 0+e],c2);patch([0 0 1 1-e 0+e 0+e],[0 1 1 1-e 1-e 0+e],c3);plot([0 1 1 0 0],[0 0 1 1 0]);
  wires:
  a/1 -> mapminmax_reverse/1
  mapminmax_reverse/1 -> y/1

== system csdesigner_Preg_14v/Subsystem9/Subsystem5/Ux ==
  Ei : Inport
  E'RPn : Inport  Port=2
  Product : Product
  Subsystem5 : Subsystem
  Ux : Outport
  wires:
  E'RPn/1 -> Product/2
  Subsystem5/1(Coefficient KP) -> Product/1
  Product/1 -> Ux/1
  Ei/1 -> Subsystem5/1(Ei1)

== system csdesigner_Preg_14v/Subsystem9/Subsystem6/Uy ==
  Ei : Inport
  E'RPn : Inport  Port=2
  Product : Product
  Scope : Scope
      settings: TimeRange=auto  MaxDataPoints=5000  SaveToWorkspace=off  SaveName=ScopeData7  YMin=-3.55043  YMax=1.33861  SampleTime=-1
  Subsystem5 : Subsystem
  Uy : Outport
  wires:
  E'RPn/1 -> Product/2
  Subsystem5/1(Coefficient KP) -> Product/1
  Product/1 -> Scope/1, Uy/1
  Ei/1 -> Subsystem5/1(Ei1)

== system csdesigner_Preg_14v/Subsystem9/Subsystem7/Ux ==
  Ei : Inport
  E'RPn : Inport  Port=2
  Product : Product
  Subsystem5 : Subsystem
  Ux : Outport
  wires:
  E'RPn/1 -> Product/2
  Subsystem5/1(Coefficient KP) -> Product/1
  Product/1 -> Ux/1
  Ei/1 -> Subsystem5/1(Ei1)

== system csdesigner_Preg_14v/Subsystem9/Subsystem8/Uy ==
  Ei : Inport
  E'RPn : Inport  Port=2
  Product : Product
  Subsystem5 : Subsystem
  Uy : Outport
  wires:
  E'RPn/1 -> Product/2
  Subsystem5/1(Coefficient KP) -> Product/1
  Product/1 -> Uy/1
  Ei/1 -> Subsystem5/1(Ei1)

== system csdesigner_Preg_14v/NONLINEAR BEARING #2 WITHOUT UNBALANCE/BEARING 2 NL/B2NN /Layer 1 ==
  "p{1}" : Inport  PortDimensions=4
      mask Display: e = 0.06;c1 = [120 230 180]/255;c2 = ([120 230 180]+0)/(256+128);c3 = ([120 230 180]+128)/(256+128);patch([0 1 1 0],[0 0 1 1],c1);patch([0 1 1 1-e 1-e 0+e],[0 0 1 1-e 0+e 0+e],c2);patch([0 0 1 1-e 0+e 0+e],[0 1 1 1-e 1-e 0+e],c3);plot([0 1 1 0 0],[0 0 1 1 0]);
  Delays 1 : Subsystem
      mask Display: e = 0.06;c1 = [120 150 230]/255;c2 = ([120 150 230]+0)/383;c3 = ([120 150 230]+128)/383;patch([0 1 1 0],[0 0 1 1],c1);patch([0 1 1 1-e 1-e 0+e],[0 0 1 1-e 0+e 0+e],c2);patch([0 0 1 1-e 0+e 0+e],[0 1 1 1-e 1-e 0+e],c3);plot([0 1 1 0 0],[0 0 1 1 0]);disp('0');
  "IW{1,1}" : Subsystem
      mask Display: e = 0.06;c1 = [120 150 230]/255;c2 = ([120 150 230]+0)/383;c3 = ([120 150 230]+128)/383;patch([0 1 1 0],[0 0 1 1],c1);patch([0 1 1 1-e 1-e 0+e],[0 0 1 1-e 0+e 0+e],c2);patch([0 0 1 1-e 0+e 0+e],[0 1 1 1-e 1-e 0+e],c3);plot([0 1 1 0 0],[0 0 1 1 0]);disp('W');
  "b{1}" : Constant  Value=[-0.2178309078748878191422733152649016119539737701416015625;-0.4663688232922715837247551462496630847454071044921875;1.0291205948709640782823271365487016737461090087890625;0.480309902987716530464723518889513798058032989501953125;1.161844801131203919197787399752996861934661865234375;-1.512967482361870619200772125623188912868499755859375;-0.273412838485520948150764297679415903985500335693359375;-0.94217390855659821635725847954745404422283172607421875;-0.07605758756975593282145808871064218692481517791748046875;-0.399790157521881794888685135447303764522075653076171875;0.79195210623637846136801954344264231622219085693359375;-3.192656660610529772981180940405465662479400634765625;-2.461688084332111170482448869734071195125579833984375;-0.1367343681641355335187881792080588638782501220703125;1.017505537075550581249672177364118397235870361328125;-2.093654754086606839535988910938613116741180419921875;0.9581022805738912406781082609086297452449798583984375;0.56402388946102177680330669318209402263164520263671875;0.71526576502755567776858924844418652355670928955078125;-0.91024327424186524115867769069154746830463409423828125;-0.70390847618132668106483151859720237553119659423828125;-4.40897960553333945199483423493802547454833984375;-2.973713982227526475554668650147505104541778564453125;1.0482416675917829440578543653828091919422149658203125;0.317549551932251372665660937855136580765247344970703125;0.731530098548386575885160709731280803680419921875;-2.675170120542511131844776173238642513751983642578125;1.8103766278381219212434416476753540337085723876953125;1.158265961724864734350148864905349910259246826171875;1.944688696809947714427835308015346527099609375;0.4034223551320514911111558831180445849895477294921875;0.0281655182581152345455688390529758180491626262664794921875;-0.150221987955851954410491089220158755779266357421875;-1.9341068217772769965989709817222319543361663818359375;-1.0238343643759808543336475850082933902740478515625;0.221748334588854678628422334440983831882476806640625;-0.9388198197484880491714420713833533227443695068359375;-2.0679451010865168569807792664505541324615478515625;-1.368368974507848445654190072673372924327850341796875;-2.735276600025368765045641339384019374847412109375;1.84503386751565212620107558905147016048431396484375;0.740345853366948691842708285548724234104156494140625;-0.5247589359035356171290231941384263336658477783203125;-1.56490918196444273036149752442725002765655517578125;0.63995198035091560573306423975736834108829498291015625;1.3379300699480338732172413074295036494731903076171875;-0.210387878801505279202643805547268129885196685791015625;2.797896808136826951596276558120734989643096923828125;-2.488271296185179171089885130641050636768341064453125;2.51543430575473525578900080290623009204864501953125;7.9013425365337486283578982693143188953399658203125;-0.470177644552810580780288773894426412880420684814453125;-2.0801539730077234224836502107791602611541748046875;2.062741497946209090486036075162701308727264404296875;-0.32071153368788285487056555211893282830715179443359375;-0.283212003982637627874652253012754954397678375244140625;1.0612309102350085954213909644749946892261505126953125;-1.1105087769466706060228489150176756083965301513671875;0.67348640024102934820149357619811780750751495361328125;0.10529861901466662510440386313348426483571529388427734375;0.391260940762822417848809664064901880919933319091796875;0.801509627119028511543774584424681961536407470703125;4.22541015087345517287076290813274681568145751953125;-1.4713116481372152666295960443676449358463287353515625;-0.283086075680045734515033473144285380840301513671875;1.2571731480514269918558056815527379512786865234375;-0.214181955816110713985978009077371098101139068603515625;-0.196712129894504650362563324961229227483272552490234375;-0.10797625994168437435494212195408181287348270416259765625;-6.52930735910772686025893563055433332920074462890625;-1.059147137326928334033482315135188400745391845703125;-2.74636677995498512672156721237115561962127685546875 ...(+1555 chars)]
      mask Display: e = 0.06;c1 = [120 150 230]/255;c2 = ([120 150 230]+0)/383;c3 = ([120 150 230]+128)/383;patch([0 1 1 0],[0 0 1 1],c1);patch([0 1 1 1-e 1-e 0+e],[0 0 1 1-e 0+e 0+e],c2);patch([0 0 1 1-e 0+e 0+e],[0 1 1 1-e 1-e 0+e],c3);plot([0 1 1 0 0],[0 0 1 1 0]);disp('b');
  netsum : Sum  Inputs=2  InputSameDT=on  SaturateOnIntegerOverflow=on  OutDataTypeStr=Inherit: Same as first input
      mask Display: e = 0.06;c1 = [120 150 230]/255;c2 = ([120 150 230]+0)/383;c3 = ([120 150 230]+128)/383;patch([0 1 1 0],[0 0 1 1],c1);patch([0 1 1 1-e 1-e 0+e],[0 0 1 1-e 0+e 0+e],c2);patch([0 0 1 1-e 0+e 0+e],[0 1 1 1-e 1-e 0+e],c3);plot([0 1 1 0 0],[0 0 1 1 0]);disp('+');
  tansig : neural/Transfer Functions/tansig
  "a{1}" : Outport  InitialOutput=[0;0;0;0;0;0;0;0;0;0;0;0;0;0;0;0;0;0;0;0;0;0;0;0;0;0;0;0;0;0;0;0;0;0;0;0;0;0;0;0;0;0;0;0;0;0;0;0;0;0;0;0;0;0;0;0;0;0;0;0;0;0;0;0;0;0;0;0;0;0;0;0;0;0;0;0;0;0;0;0;0;0;0;0;0;0;0;0;0;0;0;0;0;0;0;0;0;0;0;0]
      mask Display: e = 0.06;c1 = [120 230 180]/255;c2 = ([120 230 180]+0)/(256+128);c3 = ([120 230 180]+128)/(256+128);patch([0 1 1 0],[0 0 1 1],c1);patch([0 1 1 1-e 1-e 0+e],[0 0 1 1-e 0+e 0+e],c2);patch([0 0 1 1-e 0+e 0+e],[0 1 1 1-e 1-e 0+e],c3);plot([0 1 1 0 0],[0 0 1 1 0]);
  wires:
  "p{1}"/1 -> Delays 1/1("p{1}")
  Delays 1/1("pd{1,1}") -> "IW{1,1}"/1("pd{1,1}")
  "IW{1,1}"/1("iz{1,1}") -> netsum/1
  "b{1}"/1 -> netsum/2
  netsum/1 -> tansig/1
  tansig/1 -> "a{1}"/1

== system csdesigner_Preg_14v/NONLINEAR BEARING #2 WITHOUT UNBALANCE/BEARING 2 NL/B2NN /Layer 2 ==
  "a{1} " : Inport  PortDimensions=100
      mask Display: e = 0.06;c1 = [120 230 180]/255;c2 = ([120 230 180]+0)/(256+128);c3 = ([120 230 180]+128)/(256+128);patch([0 1 1 0],[0 0 1 1],c1);patch([0 1 1 1-e 1-e 0+e],[0 0 1 1-e 0+e 0+e],c2);patch([0 0 1 1-e 0+e 0+e],[0 1 1 1-e 1-e 0+e],c3);plot([0 1 1 0 0],[0 0 1 1 0]);
  Delays 1 : Subsystem
      mask Display: e = 0.06;c1 = [120 150 230]/255;c2 = ([120 150 230]+0)/383;c3 = ([120 150 230]+128)/383;patch([0 1 1 0],[0 0 1 1],c1);patch([0 1 1 1-e 1-e 0+e],[0 0 1 1-e 0+e 0+e],c2);patch([0 0 1 1-e 0+e 0+e],[0 1 1 1-e 1-e 0+e],c3);plot([0 1 1 0 0],[0 0 1 1 0]);disp('0');
  "LW{2,1}" : Subsystem
      mask Display: e = 0.06;c1 = [120 150 230]/255;c2 = ([120 150 230]+0)/383;c3 = ([120 150 230]+128)/383;patch([0 1 1 0],[0 0 1 1],c1);patch([0 1 1 1-e 1-e 0+e],[0 0 1 1-e 0+e 0+e],c2);patch([0 0 1 1-e 0+e 0+e],[0 1 1 1-e 1-e 0+e],c3);plot([0 1 1 0 0],[0 0 1 1 0]);disp('W');
  "b{2}" : Constant  Value=[-1.024314189728581681038122042082250118255615234375;1.068525411638810762582352253957651555538177490234375]
      mask Display: e = 0.06;c1 = [120 150 230]/255;c2 = ([120 150 230]+0)/383;c3 = ([120 150 230]+128)/383;patch([0 1 1 0],[0 0 1 1],c1);patch([0 1 1 1-e 1-e 0+e],[0 0 1 1-e 0+e 0+e],c2);patch([0 0 1 1-e 0+e 0+e],[0 1 1 1-e 1-e 0+e],c3);plot([0 1 1 0 0],[0 0 1 1 0]);disp('b');
  netsum : Sum  Inputs=2  InputSameDT=on  SaturateOnIntegerOverflow=on  OutDataTypeStr=Inherit: Same as first input
      mask Display: e = 0.06;c1 = [120 150 230]/255;c2 = ([120 150 230]+0)/383;c3 = ([120 150 230]+128)/383;patch([0 1 1 0],[0 0 1 1],c1);patch([0 1 1 1-e 1-e 0+e],[0 0 1 1-e 0+e 0+e],c2);patch([0 0 1 1-e 0+e 0+e],[0 1 1 1-e 1-e 0+e],c3);plot([0 1 1 0 0],[0 0 1 1 0]);disp('+');
  purelin : neural/Transfer Functions/purelin
  "a{2}" : Outport  InitialOutput=[0;0]
      mask Display: e = 0.06;c1 = [120 230 180]/255;c2 = ([120 230 180]+0)/(256+128);c3 = ([120 230 180]+128)/(256+128);patch([0 1 1 0],[0 0 1 1],c1);patch([0 1 1 1-e 1-e 0+e],[0 0 1 1-e 0+e 0+e],c2);patch([0 0 1 1-e 0+e 0+e],[0 1 1 1-e 1-e 0+e],c3);plot([0 1 1 0 0],[0 0 1 1 0]);
  wires:
  "a{1} "/1 -> Delays 1/1("p{2}")
  Delays 1/1("pd{2,1}") -> "LW{2,1}"/1("ad{2,1}")
  "LW{2,1}"/1("lz{2,1}") -> netsum/1
  "b{2}"/1 -> netsum/2
  netsum/1 -> purelin/1
  purelin/1 -> "a{2}"/1

== system csdesigner_Preg_14v/NONLINEAR BEARING #2 WITHOUT UNBALANCE/BEARING 2 NL/B2NN /Process Input 1 ==
  x : Inport  PortDimensions=4
      mask Display: e = 0.06;c1 = [120 230 180]/255;c2 = ([120 230 180]+0)/(256+128);c3 = ([120 230 180]+128)/(256+128);patch([0 1 1 0],[0 0 1 1],c1);patch([0 1 1 1-e 1-e 0+e],[0 0 1 1-e 0+e 0+e],c2);patch([0 0 1 1-e 0+e 0+e],[0 1 1 1-e 1-e 0+e],c3);plot([0 1 1 0 0],[0 0 1 1 0]);
  mapminmax : neural/Processing Functions/mapminmax  xmin=[-538.468980108142545759619679302;-135539.545046046550851315259933;-556.942413735731065571599174291;-162352.452120847709011286497116]  xmax=[497.590366527936510010476922616;133637.874490537593374028801918;508.231506338722681448416551575;114907.634981025839806534349918]  ymin=-1  ymax=1
  p : Outport  PortDimensions=4
      mask Display: e = 0.06;c1 = [120 230 180]/255;c2 = ([120 230 180]+0)/(256+128);c3 = ([120 230 180]+128)/(256+128);patch([0 1 1 0],[0 0 1 1],c1);patch([0 1 1 1-e 1-e 0+e],[0 0 1 1-e 0+e 0+e],c2);patch([0 0 1 1-e 0+e 0+e],[0 1 1 1-e 1-e 0+e],c3);plot([0 1 1 0 0],[0 0 1 1 0]);
  wires:
  x/1 -> mapminmax/1
  mapminmax/1 -> p/1

== system csdesigner_Preg_14v/NONLINEAR BEARING #2 WITHOUT UNBALANCE/BEARING 2 NL/B2NN /Process Output 1 ==
  a : Inport  PortDimensions=2
      mask Display: e = 0.06;c1 = [120 230 180]/255;c2 = ([120 230 180]+0)/(256+128);c3 = ([120 230 180]+128)/(256+128);patch([0 1 1 0],[0 0 1 1],c1);patch([0 1 1 1-e 1-e 0+e],[0 0 1 1-e 0+e 0+e],c2);patch([0 0 1 1-e 0+e 0+e],[0 1 1 1-e 1-e 0+e],c3);plot([0 1 1 0 0],[0 0 1 1 0]);
  mapminmax_reverse : neural/Processing Functions/mapminmax_reverse  xmin=[-75.5584088466681009776948485523;-61.1450218842471571178975864314]  xmax=[73.9887561495499994634883478284;93.9188148616534164148106356151]  ymin=-1  ymax=1
  y : Outport  PortDimensions=2
      mask Display: e = 0.06;c1 = [120 230 180]/255;c2 = ([120 230 180]+0)/(256+128);c3 = ([120 230 180]+128)/(256+128);patch([0 1 1 0],[0 0 1 1],c1);patch([0 1 1 1-e 1-e 0+e],[0 0 1 1-e 0+e 0+e],c2);patch([0 0 1 1-e 0+e 0+e],[0 1 1 1-e 1-e 0+e],c3);plot([0 1 1 0 0],[0 0 1 1 0]);
  wires:
  a/1 -> mapminmax_reverse/1
  mapminmax_reverse/1 -> y/1

== system csdesigner_Preg_14v/SERVOVALVES/HYDROSTATIC FORCES APPROXIMATION/Layer 1/Delays 1 ==
  "p{1}" : Inport  PortDimensions=4
      mask Display: e = 0.06;c1 = [120 230 180]/255;c2 = ([120 230 180]+0)/(256+128);c3 = ([120 230 180]+128)/(256+128);patch([0 1 1 0],[0 0 1 1],c1);patch([0 1 1 1-e 1-e 0+e],[0 0 1 1-e 0+e 0+e],c2);patch([0 0 1 1-e 0+e 0+e],[0 1 1 1-e 1-e 0+e],c3);plot([0 1 1 0 0],[0 0 1 1 0]);
  mux : Mux  Inputs=1
      mask Display: e = 0.06;c1 = [120 150 230]/255;c2 = ([120 150 230]+0)/383;c3 = ([120 150 230]+128)/383;patch([0 1 1 0],[0 0 1 1],c1);patch([0 1 1 1-e 1-e 0+e],[0 0 1 1-e 0+e 0+e],c2);patch([0 0 1 1-e 0+e 0+e],[0 1 1 1-e 1-e 0+e],c3);plot([0 1 1 0 0],[0 0 1 1 0]);disp('Mux')
  "pd{1,1}" : Outport
      mask Display: e = 0.06;c1 = [120 230 180]/255;c2 = ([120 230 180]+0)/(256+128);c3 = ([120 230 180]+128)/(256+128);patch([0 1 1 0],[0 0 1 1],c1);patch([0 1 1 1-e 1-e 0+e],[0 0 1 1-e 0+e 0+e],c2);patch([0 0 1 1-e 0+e 0+e],[0 1 1 1-e 1-e 0+e],c3);plot([0 1 1 0 0],[0 0 1 1 0]);
  wires:
  "p{1}"/1 -> mux/1
  mux/1 -> "pd{1,1}"/1
